simulink model "inverseKinematics"  (R2015a)
settings: Solver=ode1  StartTime=0.0  StopTime=2  FixedStep=0.001  RelTol=1e-3
undefined symbols (not defined in the file or in its folder): Kd, Kp, q0
libraries: simulink x1
settings Model: Creator=Emmanuel  LastModifiedBy=Emmanuel

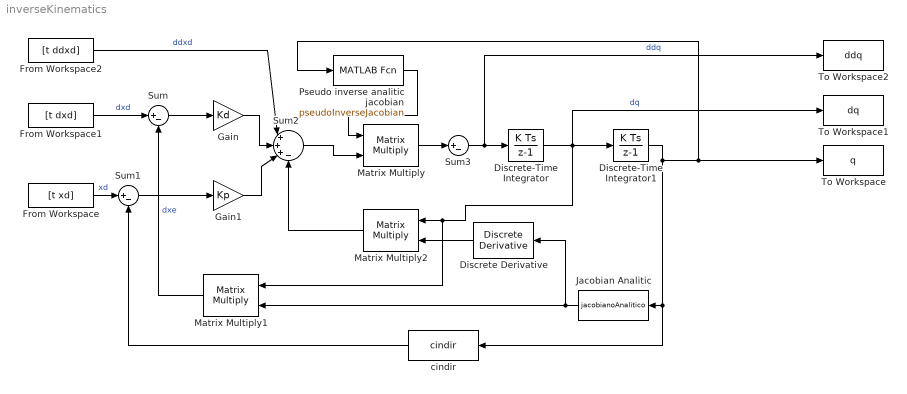
== system inverseKinematics ==
  Discrete Derivative : simulink/Discrete/Discrete Derivative  gainval=1.0  ICPrevScaledInput=0.0  InputProcessing=Inherited  OutMin=[]  OutMax=[]  OutDataType=fixdt(1, 16)  OutScaling=2^-10  DoSatur=off
  Discrete-Time Integrator : DiscreteIntegrator  InitialConditionSetting=State (most efficient)
  Discrete-Time Integrator1 : DiscreteIntegrator  InitialCondition=q0  InitialConditionSetting=State (most efficient)
  From Workspace : FromWorkspace  VariableName=[t xd]  SampleTime=0  OutputAfterFinalValue=Holding final value
  From Workspace1 : FromWorkspace  VariableName=[t dxd]  SampleTime=0  OutputAfterFinalValue=Setting to zero
  From Workspace2 : FromWorkspace  VariableName=[t ddxd]  SampleTime=0  OutputAfterFinalValue=Setting to zero
  Gain : Gain  Gain=Kd
  Gain1 : Gain  Gain=Kp
  Jacobian Analitic : MATLABFcn  MATLABFcn=jacobianoAnalitico
  Matrix Multiply : Product  Multiplication=Matrix(*)
  Matrix Multiply1 : Product  Multiplication=Matrix(*)
  Matrix Multiply2 : Product  Multiplication=Matrix(*)
  Pseudo inverse analitic jacobian : MATLABFcn  MATLABFcn=pseudoInverseJacobian
  Sum : Sum  Inputs=|+-
  Sum1 : Sum  Inputs=|+-
  Sum2 : Sum  Inputs=|+++-
  Sum3 : Sum  Inputs=|+-
  To Workspace : ToWorkspace  VariableName=q  SampleTime=-1
  To Workspace1 : ToWorkspace  VariableName=dq  SampleTime=-1
  To Workspace2 : ToWorkspace  VariableName=ddq  SampleTime=-1
  cindir : MATLABFcn  MATLABFcn=cindir
  wires:
  Sum1/1 -> Gain1/1
  Sum/1 -> Gain/1
  Gain/1 -> Sum2/2
  Gain1/1 -> Sum2/3
  Sum2/1 -> Matrix Multiply/2
  Pseudo inverse analitic jacobian/1 -> Matrix Multiply/1
  Matrix Multiply/1 -> Sum3/1
  Sum3/1 -> To Workspace2/1, Discrete-Time Integrator/1  "ddq"
  Discrete-Time Integrator/1 -> Matrix Multiply1/1, Matrix Multiply2/1, To Workspace1/1, Discrete-Time Integrator1/1  "dq"
  Jacobian Analitic/1 -> Discrete Derivative/1, Matrix Multiply1/2
  cindir/1 -> Sum1/2
  Discrete-Time Integrator1/1 -> cindir/1, Jacobian Analitic/1, Pseudo inverse analitic jacobian/1, To Workspace/1
  From Workspace1/1 -> Sum/1  "dxd"
  From Workspace/1 -> Sum1/1  "xd"
  From Workspace2/1 -> Sum2/1  "ddxd"
  Matrix Multiply1/1 -> Sum/2  "dxe"
  Discrete Derivative/1 -> Matrix Multiply2/2
  Matrix Multiply2/1 -> Sum2/4
